simulink model "Project_Sys"  (R2023b)
settings: Solver=ode23t  StartTime=0.0  StopTime=120  RelTol=1e-3
InitFcn:
  | Ts = 0.05;     % Sample time
values from neighbouring files (symbols this model uses):
  B = 4.07973550342    [Project_Dataset.mat]
  Bm = 0.00814489840092    [Project_Dataset.mat]
  g = 9.81    [Project_Dataset.mat]
  JG1 = 0.00809524979335    [Project_Dataset.mat]
  JG2 = 0.148685222339    [Project_Dataset.mat]
  Jm = 0.016692235133    [Project_Dataset.mat]
  Js1 = 0.0287642081421    [Project_Dataset.mat]
  Js2 = 0.0375031699005    [Project_Dataset.mat]
  KT = 0.696639618146    [Project_Dataset.mat]
  L = 0.270608476545    [Project_Dataset.mat]
  La = 0.0921193951949    [Project_Dataset.mat]
  m = 5.3183233869    [Project_Dataset.mat]
  N = 5    [Project_Dataset.mat]
  Ra = 14.3815472022    [Project_Dataset.mat]
libraries: fl_lib x36, nesl_utility x9, ee_lib x3
settings Model: Creator=n01356818  LastModifiedBy=Mystic

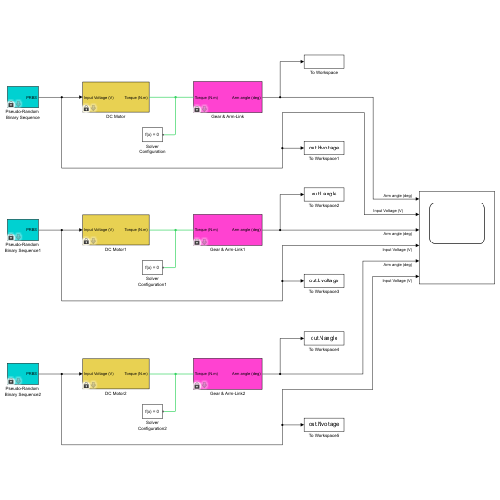
[thumbnail: Simulink's stored preview of the top-level diagram]
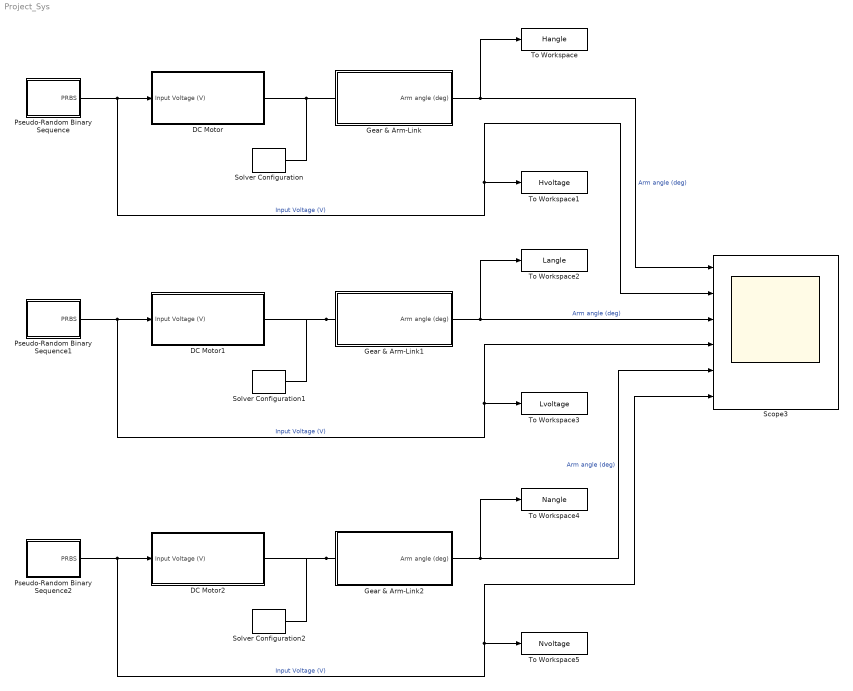
== system Project_Sys ==
  DC Motor : Subsystem  mask(DC Motor){Ra=Ra, La=La, Jm=Jm, Bm=Bm, KT=KT}
      mask prompts: Ra "Armature Resistance - Ra (ohms)"; La "Armature Inductance - La (H)"; Jm "Rotor Inertia - Jm (kg.m^2)"; Bm "Rotor Damping - Bm (N.m.s/rad)"; KT "Torque Constant - KT (N.m/A)"
      mask help: Armature-controlled permanent magnet DC motor with dead-zone nonlinearity.
  DC Motor1 : Subsystem  mask(DC Motor){Ra=Ra, La=La, Jm=Jm, Bm=Bm, KT=KT}
      mask prompts: Ra "Armature Resistance - Ra (ohms)"; La "Armature Inductance - La (H)"; Jm "Rotor Inertia - Jm (kg.m^2)"; Bm "Rotor Damping - Bm (N.m.s/rad)"; KT "Torque Constant - KT (N.m/A)"
      mask help: Armature-controlled permanent magnet DC motor with dead-zone nonlinearity.
  DC Motor2 : Subsystem  mask(DC Motor){Ra=Ra, La=La, Jm=Jm, Bm=Bm, KT=KT}
      mask prompts: Ra "Armature Resistance - Ra (ohms)"; La "Armature Inductance - La (H)"; Jm "Rotor Inertia - Jm (kg.m^2)"; Bm "Rotor Damping - Bm (N.m.s/rad)"; KT "Torque Constant - KT (N.m/A)"
      mask help: Armature-controlled permanent magnet DC motor with dead-zone nonlinearity.
  Gear & Arm-Link : Subsystem  mask(Gear and Arm-link){Js1=Js1, JG1=JG1, Js2=Js2, JG2=JG2, N=N, B=B, m=m, L=L, g=g, noise=1, Ts=Ts}
      mask prompts: Js1 "Drive-side shaft inertia - Js1 (kg.m^2)"; JG1 "Drive-side gear inertia - JG1 (kg.m^2)"; Js2 "Driven-side shaft inertia - Js2 (kg.m^2)"; JG2 "Driven-side gear inertia - JG2 (kg.m^2)"; N "Gear ratio - N (N2/N1)"; B "Damping friction of shaft and arm - B (N.m.s/rad)"; m "Arm mass - m (kg)"; L "Distance of mass center from asix of rotation - L (m)"; g "Gravitational acceleration - g (m/s^2)"; noise "Additive noise (OFF=0, ON=1)"; Ts "Sample time - Ts (sec)"
  Gear & Arm-Link1 : Subsystem  mask(Gear and Arm-link){Js1=Js1, JG1=JG1, Js2=Js2, JG2=JG2, N=N, B=B, m=m, L=L, g=g, noise=1, Ts=Ts}
      mask prompts: Js1 "Drive-side shaft inertia - Js1 (kg.m^2)"; JG1 "Drive-side gear inertia - JG1 (kg.m^2)"; Js2 "Driven-side shaft inertia - Js2 (kg.m^2)"; JG2 "Driven-side gear inertia - JG2 (kg.m^2)"; N "Gear ratio - N (N2/N1)"; B "Damping friction of shaft and arm - B (N.m.s/rad)"; m "Arm mass - m (kg)"; L "Distance of mass center from asix of rotation - L (m)"; g "Gravitational acceleration - g (m/s^2)"; noise "Additive noise (OFF=0, ON=1)"; Ts "Sample time - Ts (sec)"
  Gear & Arm-Link2 : Subsystem  mask(Gear and Arm-link){Js1=Js1, JG1=JG1, Js2=Js2, JG2=JG2, N=N, B=B, m=m, L=L, g=g, noise=0, Ts=Ts}
      mask prompts: Js1 "Drive-side shaft inertia - Js1 (kg.m^2)"; JG1 "Drive-side gear inertia - JG1 (kg.m^2)"; Js2 "Driven-side shaft inertia - Js2 (kg.m^2)"; JG2 "Driven-side gear inertia - JG2 (kg.m^2)"; N "Gear ratio - N (N2/N1)"; B "Damping friction of shaft and arm - B (N.m.s/rad)"; m "Arm mass - m (kg)"; L "Distance of mass center from asix of rotation - L (m)"; g "Gravitational acceleration - g (m/s^2)"; noise "Additive noise (OFF=0, ON=1)"; Ts "Sample time - Ts (sec)"
  Pseudo-Random Binary Sequence : Subsystem  mask(DPRBS){N=250, K=200, A=24}
      mask prompts: N "Number of Sample Points (N)"; K "Switch Constant (K)"; A "Amplitude (A)"
      mask help: Generates a random switching sequence of discrete samples valued at -A and +A.
  Pseudo-Random Binary Sequence1 : Subsystem  mask(DPRBS){N=250, K=200, A=9}
      mask prompts: N "Number of Sample Points (N)"; K "Switch Constant (K)"; A "Amplitude (A)"
      mask help: Generates a random switching sequence of discrete samples valued at -A and +A.
  Pseudo-Random Binary Sequence2 : Subsystem  mask(DPRBS){N=250, K=200, A=24}
      mask prompts: N "Number of Sample Points (N)"; K "Switch Constant (K)"; A "Amplitude (A)"
      mask help: Generates a random switching sequence of discrete samples valued at -A and +A.
  Scope3 : Scope  NumInputPorts=6
  Solver Configuration : nesl_utility/Solver Configuration  PhysicalDomain=network_engine_domain  SubClassName=solver  LeftPortType=input  RightPortType=generic  Tones=[]  Harmonics=[]  SimulateNoise=off  Profile=off  UseLocalSampling=off  EnableSwitchedLinearOptims=on  FrequencyDomain=off  UseCCode=off  RelTol=0.001  AbsTol=0.001  MinStep=1e-09  ToWorkspace=off  RevertToSquareIcSolve=off  NumHomotopyIterations=100  PhasorMode=off  PhasorModeNumHarmonics=1  ConsistencySolver=NEWTON_XTOL_AFTER_FTOL  IndexReductionMethod=DerivativeReplacement  DoDC=off  ResidualTolerance=1e-09  ConsistencyTolSource=GLOBAL  ConsistencyAbsTol=0.001  ConsistencyRelTol=0.001  ConsistencyTolFactor=0.001  UseLocalSolver=off  LocalSolverChoice=NE_BACKWARD_EULER_ADVANCER  ResolveIndetEquations=on  FunctionEvalNumThread=1  LocalSolverSampleTime=0.001  DoFixedCost=off  MaxNonlinIter=3  MaxModeIter=2  ComputeImpulses=off  ImpulseIterations=2  LinearAlgebra=auto  LinearAlgebraNumThread=0  EquationFormulation=NE_TIME_EF  DelaysMemoryBudget=1024  AutomaticFiltering=on  FilteringTimeConstant=0.001  PartitionStorageMethod=AS_NEEDED  PartitionMemoryBudget=1024  PartitionMethod=ROBUST  MultibodyUseLocalSolver=off  MultibodyLocalSolverChoice=ODE1  MultibodyLocalSolverSampleTime=0.001
  Solver Configuration1 : nesl_utility/Solver Configuration  PhysicalDomain=network_engine_domain  SubClassName=solver  LeftPortType=input  RightPortType=generic  Tones=[]  Harmonics=[]  SimulateNoise=off  Profile=off  UseLocalSampling=off  EnableSwitchedLinearOptims=on  FrequencyDomain=off  UseCCode=off  RelTol=0.001  AbsTol=0.001  MinStep=1e-09  ToWorkspace=off  RevertToSquareIcSolve=off  NumHomotopyIterations=100  PhasorMode=off  PhasorModeNumHarmonics=1  ConsistencySolver=NEWTON_XTOL_AFTER_FTOL  IndexReductionMethod=DerivativeReplacement  DoDC=off  ResidualTolerance=1e-09  ConsistencyTolSource=GLOBAL  ConsistencyAbsTol=0.001  ConsistencyRelTol=0.001  ConsistencyTolFactor=0.001  UseLocalSolver=off  LocalSolverChoice=NE_BACKWARD_EULER_ADVANCER  ResolveIndetEquations=on  FunctionEvalNumThread=1  LocalSolverSampleTime=0.001  DoFixedCost=off  MaxNonlinIter=3  MaxModeIter=2  ComputeImpulses=off  ImpulseIterations=2  LinearAlgebra=auto  LinearAlgebraNumThread=0  EquationFormulation=NE_TIME_EF  DelaysMemoryBudget=1024  AutomaticFiltering=on  FilteringTimeConstant=0.001  PartitionStorageMethod=AS_NEEDED  PartitionMemoryBudget=1024  PartitionMethod=ROBUST  MultibodyUseLocalSolver=off  MultibodyLocalSolverChoice=ODE1  MultibodyLocalSolverSampleTime=0.001
  Solver Configuration2 : nesl_utility/Solver Configuration  PhysicalDomain=network_engine_domain  SubClassName=solver  LeftPortType=input  RightPortType=generic  Tones=[]  Harmonics=[]  SimulateNoise=off  Profile=off  UseLocalSampling=off  EnableSwitchedLinearOptims=on  FrequencyDomain=off  UseCCode=off  RelTol=0.001  AbsTol=0.001  MinStep=1e-09  ToWorkspace=off  RevertToSquareIcSolve=off  NumHomotopyIterations=100  PhasorMode=off  PhasorModeNumHarmonics=1  ConsistencySolver=NEWTON_XTOL_AFTER_FTOL  IndexReductionMethod=DerivativeReplacement  DoDC=off  ResidualTolerance=1e-09  ConsistencyTolSource=GLOBAL  ConsistencyAbsTol=0.001  ConsistencyRelTol=0.001  ConsistencyTolFactor=0.001  UseLocalSolver=off  LocalSolverChoice=NE_BACKWARD_EULER_ADVANCER  ResolveIndetEquations=on  FunctionEvalNumThread=1  LocalSolverSampleTime=0.001  DoFixedCost=off  MaxNonlinIter=3  MaxModeIter=2  ComputeImpulses=off  ImpulseIterations=2  LinearAlgebra=auto  LinearAlgebraNumThread=0  EquationFormulation=NE_TIME_EF  DelaysMemoryBudget=1024  AutomaticFiltering=on  FilteringTimeConstant=0.001  PartitionStorageMethod=AS_NEEDED  PartitionMemoryBudget=1024  PartitionMethod=ROBUST  MultibodyUseLocalSolver=off  MultibodyLocalSolverChoice=ODE1  MultibodyLocalSolverSampleTime=0.001
  To Workspace : ToWorkspace  VariableName=Hangle  SampleTime=Ts
  To Workspace1 : ToWorkspace  VariableName=Hvoltage  SampleTime=Ts
  To Workspace2 : ToWorkspace  VariableName=Langle  SampleTime=Ts
  To Workspace3 : ToWorkspace  VariableName=Lvoltage  SampleTime=Ts
  To Workspace4 : ToWorkspace  VariableName=Nangle  SampleTime=Ts
  To Workspace5 : ToWorkspace  VariableName=Nvoltage  SampleTime=Ts
  wires:
  Pseudo-Random Binary Sequence/1(PRBS) -> Scope3/2, To Workspace1/1, DC Motor/1(Input Voltage (V))  "Input Voltage (V)"
  Gear & Arm-Link/1(Arm angle (deg)) -> Scope3/1, To Workspace/1  "Arm angle (deg)"
  Pseudo-Random Binary Sequence1/1(PRBS) -> Scope3/4, To Workspace3/1, DC Motor1/1(Input Voltage (V))  "Input Voltage (V)"
  Gear & Arm-Link1/1(Arm angle (deg)) -> Scope3/3, To Workspace2/1  "Arm angle (deg)"
  Pseudo-Random Binary Sequence2/1(PRBS) -> Scope3/6, To Workspace5/1, DC Motor2/1(Input Voltage (V))  "Input Voltage (V)"
  Gear & Arm-Link2/1(Arm angle (deg)) -> Scope3/5, To Workspace4/1  "Arm angle (deg)"
  connections:
  DC Motor/RConn1 -- Solver Configuration/RConn1 -- Gear & Arm-Link/LConn1
  Gear & Arm-Link1/LConn1 -- DC Motor1/RConn1 -- Solver Configuration1/RConn1
  Gear & Arm-Link2/LConn1 -- DC Motor2/RConn1 -- Solver Configuration2/RConn1

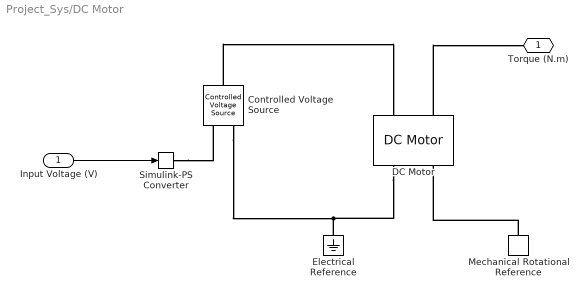
== system Project_Sys/DC Motor ==
  Input Voltage (V) : Inport
  Controlled Voltage Source : fl_lib/Electrical/Electrical Sources/Controlled Voltage Source
  DC Motor : ee_lib/Electromechanical/Brushed Motors/DC Motor  field_option=ee.enum.field_option.pm  Rf=100 Ohm  Lf=1 H  Laf=0.15 H  If0=0 A  parameterization=ee.enum.dcparam_option.circuit_param  Ra=Ra Ohm  La=La H  emf_or_torque=ee.enum.emf_or_torque.ki  Kv=0.4 V*s/rad  Ki=KT N*m/A  T_stall=0.24e-3 N*m  w_max=19100 rpm  w_rated=15000 rpm  P_rated=0.08 W  V_rated=1.5 V  lam_param=ee.enum.lam_param.damping  i_noload=0 A  V_i_noload=1.5 V  J=Jm kg*m^2  lam=Bm N*m*s/rad  speed0=0 rpm  enable_fault_armature=simscape.enum.onoff.off  rev_faulted=1 / 3  G_faulted_armature=1e-5 S  fault_trigger_armature=ee.enum.faults.faultTrigger.temporal  t_fault_armature=1 s  max_permissible_current_armature=inf A  t_fail_on_current_armature=1 s  enable_fault_field=simscape.enum.onoff.off  G_faulted_field=1e-5 S  fault_trigger_field=ee.enum.faults.faultTrigger.temporal  t_fault_field=1 s  max_permissible_current_field=inf A  t_fail_on_current_field=1 s  fault_action=simscape.enum.assert.action.none  alpha=3.93e-3 1/K  Tmeas=25 degC  thermal_mass=100 J/K  initial_temperature=25 degC
  Electrical Reference : fl_lib/Electrical/Electrical Elements/Electrical Reference
  Mechanical Rotational Reference : fl_lib/Mechanical/Rotational Elements/Mechanical Rotational Reference
  Simulink-PS Converter : nesl_utility/Simulink-PS Converter  PhysicalDomain=network_engine_domain  SubClassName=ps_input  LeftPortType=input  RightPortType=output  PseudoPeriodic=off  Frequencies=[]  NoiseDistribution=none  NoiseParameters=[]  Unit=1  AffineConversion=off  FilteringAndDerivatives=provide  SimscapeFilterOrder=1  InputFilterTimeConstant=0.001  UdotUserProvided=0
  Torque (N.m) : PMIOPort  Side=Right
  wires:
  Input Voltage (V)/1 -> Simulink-PS Converter/1
  connections:
  DC Motor/RConn1 -- Controlled Voltage Source/RConn2 -- Electrical Reference/LConn1
  Simulink-PS Converter/RConn1 -- Controlled Voltage Source/RConn1
  Controlled Voltage Source/LConn1 -- DC Motor/LConn1
  Mechanical Rotational Reference/LConn1 -- DC Motor/RConn2
  DC Motor/LConn2 -- Torque (N.m)/RConn1

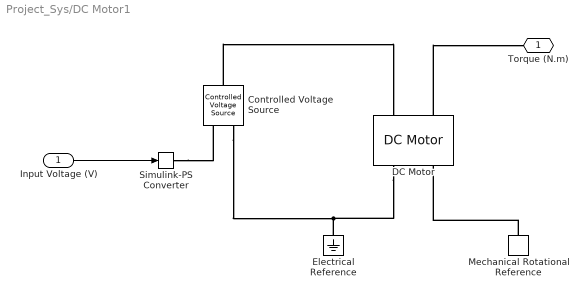
== system Project_Sys/DC Motor1 ==
  Input Voltage (V) : Inport
  Controlled Voltage Source : fl_lib/Electrical/Electrical Sources/Controlled Voltage Source
  DC Motor : ee_lib/Electromechanical/Brushed Motors/DC Motor  field_option=ee.enum.field_option.pm  Rf=100 Ohm  Lf=1 H  Laf=0.15 H  If0=0 A  parameterization=ee.enum.dcparam_option.circuit_param  Ra=Ra Ohm  La=La H  emf_or_torque=ee.enum.emf_or_torque.ki  Kv=0.4 V*s/rad  Ki=KT N*m/A  T_stall=0.24e-3 N*m  w_max=19100 rpm  w_rated=15000 rpm  P_rated=0.08 W  V_rated=1.5 V  lam_param=ee.enum.lam_param.damping  i_noload=0 A  V_i_noload=1.5 V  J=Jm kg*m^2  lam=Bm N*m*s/rad  speed0=0 rpm  enable_fault_armature=simscape.enum.onoff.off  rev_faulted=1 / 3  G_faulted_armature=1e-5 S  fault_trigger_armature=ee.enum.faults.faultTrigger.temporal  t_fault_armature=1 s  max_permissible_current_armature=inf A  t_fail_on_current_armature=1 s  enable_fault_field=simscape.enum.onoff.off  G_faulted_field=1e-5 S  fault_trigger_field=ee.enum.faults.faultTrigger.temporal  t_fault_field=1 s  max_permissible_current_field=inf A  t_fail_on_current_field=1 s  fault_action=simscape.enum.assert.action.none  alpha=3.93e-3 1/K  Tmeas=25 degC  thermal_mass=100 J/K  initial_temperature=25 degC
  Electrical Reference : fl_lib/Electrical/Electrical Elements/Electrical Reference
  Mechanical Rotational Reference : fl_lib/Mechanical/Rotational Elements/Mechanical Rotational Reference
  Simulink-PS Converter : nesl_utility/Simulink-PS Converter  PhysicalDomain=network_engine_domain  SubClassName=ps_input  LeftPortType=input  RightPortType=output  PseudoPeriodic=off  Frequencies=[]  NoiseDistribution=none  NoiseParameters=[]  Unit=1  AffineConversion=off  FilteringAndDerivatives=provide  SimscapeFilterOrder=1  InputFilterTimeConstant=0.001  UdotUserProvided=0
  Torque (N.m) : PMIOPort  Side=Right
  wires:
  Input Voltage (V)/1 -> Simulink-PS Converter/1
  connections:
  DC Motor/RConn1 -- Controlled Voltage Source/RConn2 -- Electrical Reference/LConn1
  Simulink-PS Converter/RConn1 -- Controlled Voltage Source/RConn1
  Controlled Voltage Source/LConn1 -- DC Motor/LConn1
  Mechanical Rotational Reference/LConn1 -- DC Motor/RConn2
  DC Motor/LConn2 -- Torque (N.m)/RConn1

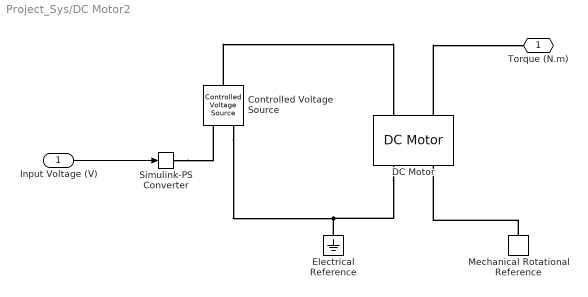
== system Project_Sys/DC Motor2 ==
  Input Voltage (V) : Inport
  Controlled Voltage Source : fl_lib/Electrical/Electrical Sources/Controlled Voltage Source
  DC Motor : ee_lib/Electromechanical/Brushed Motors/DC Motor  field_option=ee.enum.field_option.pm  Rf=100 Ohm  Lf=1 H  Laf=0.15 H  If0=0 A  parameterization=ee.enum.dcparam_option.circuit_param  Ra=Ra Ohm  La=La H  emf_or_torque=ee.enum.emf_or_torque.ki  Kv=0.4 V*s/rad  Ki=KT N*m/A  T_stall=0.24e-3 N*m  w_max=19100 rpm  w_rated=15000 rpm  P_rated=0.08 W  V_rated=1.5 V  lam_param=ee.enum.lam_param.damping  i_noload=0 A  V_i_noload=1.5 V  J=Jm kg*m^2  lam=Bm N*m*s/rad  speed0=0 rpm  enable_fault_armature=simscape.enum.onoff.off  rev_faulted=1 / 3  G_faulted_armature=1e-5 S  fault_trigger_armature=ee.enum.faults.faultTrigger.temporal  t_fault_armature=1 s  max_permissible_current_armature=inf A  t_fail_on_current_armature=1 s  enable_fault_field=simscape.enum.onoff.off  G_faulted_field=1e-5 S  fault_trigger_field=ee.enum.faults.faultTrigger.temporal  t_fault_field=1 s  max_permissible_current_field=inf A  t_fail_on_current_field=1 s  fault_action=simscape.enum.assert.action.none  alpha=3.93e-3 1/K  Tmeas=25 degC  thermal_mass=100 J/K  initial_temperature=25 degC
  Electrical Reference : fl_lib/Electrical/Electrical Elements/Electrical Reference
  Mechanical Rotational Reference : fl_lib/Mechanical/Rotational Elements/Mechanical Rotational Reference
  Simulink-PS Converter : nesl_utility/Simulink-PS Converter  PhysicalDomain=network_engine_domain  SubClassName=ps_input  LeftPortType=input  RightPortType=output  PseudoPeriodic=off  Frequencies=[]  NoiseDistribution=none  NoiseParameters=[]  Unit=1  AffineConversion=off  FilteringAndDerivatives=provide  SimscapeFilterOrder=1  InputFilterTimeConstant=0.001  UdotUserProvided=0
  Torque (N.m) : PMIOPort  Side=Right
  wires:
  Input Voltage (V)/1 -> Simulink-PS Converter/1
  connections:
  DC Motor/RConn1 -- Controlled Voltage Source/RConn2 -- Electrical Reference/LConn1
  Simulink-PS Converter/RConn1 -- Controlled Voltage Source/RConn1
  Controlled Voltage Source/LConn1 -- DC Motor/LConn1
  Mechanical Rotational Reference/LConn1 -- DC Motor/RConn2
  DC Motor/LConn2 -- Torque (N.m)/RConn1

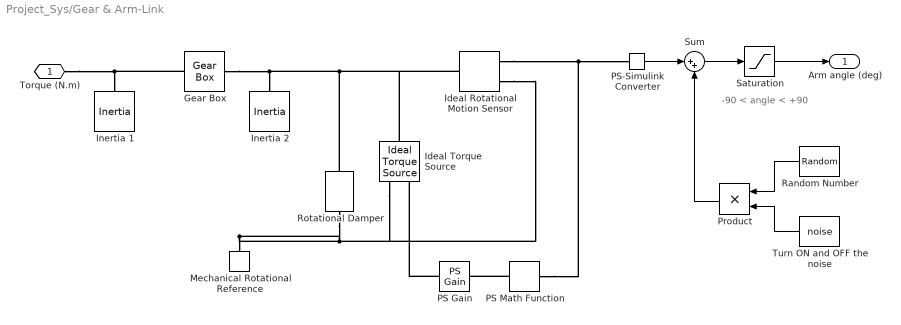
== system Project_Sys/Gear & Arm-Link ==
  note: -90 < angle < +90
  Gear Box : fl_lib/Mechanical/Mechanisms/Gear Box  ratio=N  t_in_specify=off  t_in_priority=None  t_in=0 N*m  t_in_nominal_specify=off  t_in_nominal_unit=N*m  t_in_nominal_value=1  t_out_specify=off  t_out_priority=None  t_out=0 N*m  t_out_nominal_specify=off  t_out_nominal_unit=N*m  t_out_nominal_value=1
  Ideal Rotational Motion Sensor : fl_lib/Mechanical/Mechanical Sensors/Ideal Rotational Motion Sensor  reference=foundation.enum.MeasurementReference.difference  acceleration_port=false  velocity_port=false  position_port=true  wrap_angle=false  offset=0 rad
      settings: InternalSimscapePortConfiguration="{\"Bottom\":[],\"Left\":[{\"id\":\"R\",\"label\":\"R\",\"type\":\"foundation.mechanical.rotational.rotational\"}],\"Right\":[{\"id\":\"C\",\"label\":\"C\",\"type\":\"foundation.mechanical.rotational.rotational\"},{\"id\":\"A\",\"label\":\"A\",\"type\":\"output\"}],\"Top\":[]}"
  Ideal Torque Source : fl_lib/Mechanical/Mechanical Sources/Ideal Torque Source
  Inertia 1 : fl_lib/Mechanical/Rotational Elements/Inertia  inertia=Js1+JG1 kg*m^2  num_ports=foundation.enum.numPorts2.one  w_specify=off  w_priority=High  w=0 rad/s  w_nominal_specify=off  w_nominal_unit=rad/s  w_nominal_value=1  t_specify=off  t_priority=None  t=0 N*m  t_nominal_specify=off  t_nominal_unit=N*m  t_nominal_value=1
  Inertia 2 : fl_lib/Mechanical/Rotational Elements/Inertia  inertia=Js2+JG2 kg*m^2  num_ports=foundation.enum.numPorts2.one  w_specify=off  w_priority=High  w=0 rad/s  w_nominal_specify=off  w_nominal_unit=rad/s  w_nominal_value=1  t_specify=off  t_priority=None  t=0 N*m  t_nominal_specify=off  t_nominal_unit=N*m  t_nominal_value=1
  Mechanical Rotational Reference : fl_lib/Mechanical/Rotational Elements/Mechanical Rotational Reference
  PS Gain : fl_lib/Physical Signals/Functions/PS Gain  gain=-m*g*L
  PS Math Function : fl_lib/Physical Signals/Functions/PS Math Function  fcn_choice=foundation.enum.math_function.sin  v=1
  PS-Simulink Converter : nesl_utility/PS-Simulink Converter  PhysicalDomain=network_engine_domain  SubClassName=ps_output  LeftPortType=input  RightPortType=output  PseudoPeriodic=off  Frequencies=[]  VectorFormat=inherit  Unit=deg  AffineConversion=off
  Product : Product
  Random Number : RandomNumber  Seed=randi([0 100],1,1)  SampleTime=0.1*Ts
  Rotational Damper : fl_lib/Mechanical/Rotational Elements/Rotational Damper  D=B N*m*s/rad  w_specify=off  w_priority=None  w=0 rad/s  w_nominal_specify=off  w_nominal_unit=rad/s  w_nominal_value=1  t_specify=off  t_priority=None  t=0 N*m  t_nominal_specify=off  t_nominal_unit=N*m  t_nominal_value=1
  Saturation : Saturate  UpperLimit=90  LowerLimit=-90
  Sum : Sum  Inputs=|++
  Turn ON and OFF the noise : Constant  Value=noise  SampleTime=0.1*Ts
  Torque (N.m) : PMIOPort  Side=Left
  Arm angle (deg) : Outport
  wires:
  Turn ON and OFF the noise/1 -> Product/2
  Random Number/1 -> Product/1
  Product/1 -> Sum/2
  PS-Simulink Converter/1 -> Sum/1
  Sum/1 -> Saturation/1
  Saturation/1 -> Arm angle (deg)/1
  connections:
  PS Gain/RConn1 -- Ideal Torque Source/RConn1
  Ideal Rotational Motion Sensor/RConn2 -- PS Math Function/LConn1 -- PS-Simulink Converter/LConn1
  Mechanical Rotational Reference/LConn1 -- Ideal Rotational Motion Sensor/RConn1 -- Ideal Torque Source/RConn2 -- Rotational Damper/RConn1
  PS Math Function/RConn1 -- PS Gain/LConn1
  Gear Box/RConn1 -- Ideal Rotational Motion Sensor/LConn1 -- Ideal Torque Source/LConn1 -- Rotational Damper/LConn1 -- Inertia 2/LConn1
  Gear Box/LConn1 -- Torque (N.m)/RConn1 -- Inertia 1/LConn1

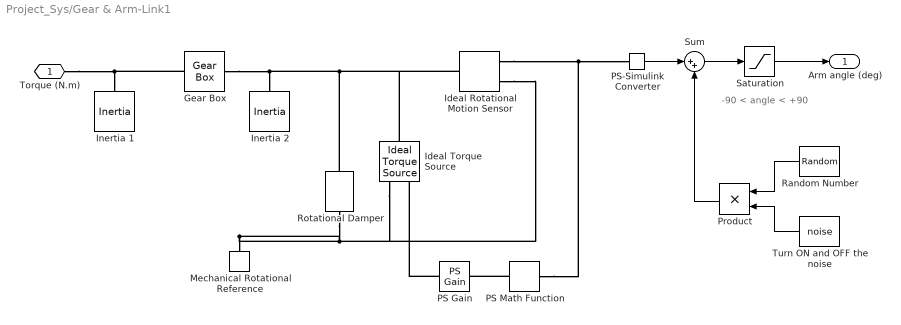
== system Project_Sys/Gear & Arm-Link1 ==
  note: -90 < angle < +90
  Gear Box : fl_lib/Mechanical/Mechanisms/Gear Box  ratio=N  t_in_specify=off  t_in_priority=None  t_in=0 N*m  t_in_nominal_specify=off  t_in_nominal_unit=N*m  t_in_nominal_value=1  t_out_specify=off  t_out_priority=None  t_out=0 N*m  t_out_nominal_specify=off  t_out_nominal_unit=N*m  t_out_nominal_value=1
  Ideal Rotational Motion Sensor : fl_lib/Mechanical/Mechanical Sensors/Ideal Rotational Motion Sensor  reference=foundation.enum.MeasurementReference.difference  acceleration_port=false  velocity_port=false  position_port=true  wrap_angle=false  offset=0 rad
      settings: InternalSimscapePortConfiguration="{\"Bottom\":[],\"Left\":[{\"id\":\"R\",\"label\":\"R\",\"type\":\"foundation.mechanical.rotational.rotational\"}],\"Right\":[{\"id\":\"C\",\"label\":\"C\",\"type\":\"foundation.mechanical.rotational.rotational\"},{\"id\":\"A\",\"label\":\"A\",\"type\":\"output\"}],\"Top\":[]}"
  Ideal Torque Source : fl_lib/Mechanical/Mechanical Sources/Ideal Torque Source
  Inertia 1 : fl_lib/Mechanical/Rotational Elements/Inertia  inertia=Js1+JG1 kg*m^2  num_ports=foundation.enum.numPorts2.one  w_specify=off  w_priority=High  w=0 rad/s  w_nominal_specify=off  w_nominal_unit=rad/s  w_nominal_value=1  t_specify=off  t_priority=None  t=0 N*m  t_nominal_specify=off  t_nominal_unit=N*m  t_nominal_value=1
  Inertia 2 : fl_lib/Mechanical/Rotational Elements/Inertia  inertia=Js2+JG2 kg*m^2  num_ports=foundation.enum.numPorts2.one  w_specify=off  w_priority=High  w=0 rad/s  w_nominal_specify=off  w_nominal_unit=rad/s  w_nominal_value=1  t_specify=off  t_priority=None  t=0 N*m  t_nominal_specify=off  t_nominal_unit=N*m  t_nominal_value=1
  Mechanical Rotational Reference : fl_lib/Mechanical/Rotational Elements/Mechanical Rotational Reference
  PS Gain : fl_lib/Physical Signals/Functions/PS Gain  gain=-m*g*L
  PS Math Function : fl_lib/Physical Signals/Functions/PS Math Function  fcn_choice=foundation.enum.math_function.sin  v=1
  PS-Simulink Converter : nesl_utility/PS-Simulink Converter  PhysicalDomain=network_engine_domain  SubClassName=ps_output  LeftPortType=input  RightPortType=output  PseudoPeriodic=off  Frequencies=[]  VectorFormat=inherit  Unit=deg  AffineConversion=off
  Product : Product
  Random Number : RandomNumber  Seed=randi([0 100],1,1)  SampleTime=0.1*Ts
  Rotational Damper : fl_lib/Mechanical/Rotational Elements/Rotational Damper  D=B N*m*s/rad  w_specify=off  w_priority=None  w=0 rad/s  w_nominal_specify=off  w_nominal_unit=rad/s  w_nominal_value=1  t_specify=off  t_priority=None  t=0 N*m  t_nominal_specify=off  t_nominal_unit=N*m  t_nominal_value=1
  Saturation : Saturate  UpperLimit=90  LowerLimit=-90
  Sum : Sum  Inputs=|++
  Turn ON and OFF the noise : Constant  Value=noise  SampleTime=0.1*Ts
  Torque (N.m) : PMIOPort  Side=Left
  Arm angle (deg) : Outport
  wires:
  Turn ON and OFF the noise/1 -> Product/2
  Random Number/1 -> Product/1
  Product/1 -> Sum/2
  PS-Simulink Converter/1 -> Sum/1
  Sum/1 -> Saturation/1
  Saturation/1 -> Arm angle (deg)/1
  connections:
  PS Gain/RConn1 -- Ideal Torque Source/RConn1
  Ideal Rotational Motion Sensor/RConn2 -- PS Math Function/LConn1 -- PS-Simulink Converter/LConn1
  Mechanical Rotational Reference/LConn1 -- Ideal Rotational Motion Sensor/RConn1 -- Ideal Torque Source/RConn2 -- Rotational Damper/RConn1
  PS Math Function/RConn1 -- PS Gain/LConn1
  Gear Box/RConn1 -- Ideal Rotational Motion Sensor/LConn1 -- Ideal Torque Source/LConn1 -- Rotational Damper/LConn1 -- Inertia 2/LConn1
  Gear Box/LConn1 -- Torque (N.m)/RConn1 -- Inertia 1/LConn1

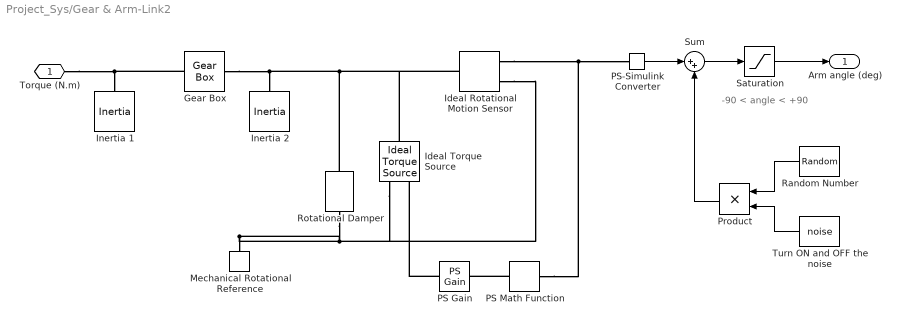
== system Project_Sys/Gear & Arm-Link2 ==
  note: -90 < angle < +90
  Gear Box : fl_lib/Mechanical/Mechanisms/Gear Box  ratio=N  t_in_specify=off  t_in_priority=None  t_in=0 N*m  t_in_nominal_specify=off  t_in_nominal_unit=N*m  t_in_nominal_value=1  t_out_specify=off  t_out_priority=None  t_out=0 N*m  t_out_nominal_specify=off  t_out_nominal_unit=N*m  t_out_nominal_value=1
  Ideal Rotational Motion Sensor : fl_lib/Mechanical/Mechanical Sensors/Ideal Rotational Motion Sensor  reference=foundation.enum.MeasurementReference.difference  acceleration_port=false  velocity_port=false  position_port=true  wrap_angle=false  offset=0 rad
      settings: InternalSimscapePortConfiguration="{\"Bottom\":[],\"Left\":[{\"id\":\"R\",\"label\":\"R\",\"type\":\"foundation.mechanical.rotational.rotational\"}],\"Right\":[{\"id\":\"C\",\"label\":\"C\",\"type\":\"foundation.mechanical.rotational.rotational\"},{\"id\":\"A\",\"label\":\"A\",\"type\":\"output\"}],\"Top\":[]}"
  Ideal Torque Source : fl_lib/Mechanical/Mechanical Sources/Ideal Torque Source
  Inertia 1 : fl_lib/Mechanical/Rotational Elements/Inertia  inertia=Js1+JG1 kg*m^2  num_ports=foundation.enum.numPorts2.one  w_specify=off  w_priority=High  w=0 rad/s  w_nominal_specify=off  w_nominal_unit=rad/s  w_nominal_value=1  t_specify=off  t_priority=None  t=0 N*m  t_nominal_specify=off  t_nominal_unit=N*m  t_nominal_value=1
  Inertia 2 : fl_lib/Mechanical/Rotational Elements/Inertia  inertia=Js2+JG2 kg*m^2  num_ports=foundation.enum.numPorts2.one  w_specify=off  w_priority=High  w=0 rad/s  w_nominal_specify=off  w_nominal_unit=rad/s  w_nominal_value=1  t_specify=off  t_priority=None  t=0 N*m  t_nominal_specify=off  t_nominal_unit=N*m  t_nominal_value=1
  Mechanical Rotational Reference : fl_lib/Mechanical/Rotational Elements/Mechanical Rotational Reference
  PS Gain : fl_lib/Physical Signals/Functions/PS Gain  gain=-m*g*L
  PS Math Function : fl_lib/Physical Signals/Functions/PS Math Function  fcn_choice=foundation.enum.math_function.sin  v=1
  PS-Simulink Converter : nesl_utility/PS-Simulink Converter  PhysicalDomain=network_engine_domain  SubClassName=ps_output  LeftPortType=input  RightPortType=output  PseudoPeriodic=off  Frequencies=[]  VectorFormat=inherit  Unit=deg  AffineConversion=off
  Product : Product
  Random Number : RandomNumber  Seed=randi([0 100],1,1)  SampleTime=0.1*Ts
  Rotational Damper : fl_lib/Mechanical/Rotational Elements/Rotational Damper  D=B N*m*s/rad  w_specify=off  w_priority=None  w=0 rad/s  w_nominal_specify=off  w_nominal_unit=rad/s  w_nominal_value=1  t_specify=off  t_priority=None  t=0 N*m  t_nominal_specify=off  t_nominal_unit=N*m  t_nominal_value=1
  Saturation : Saturate  UpperLimit=90  LowerLimit=-90
  Sum : Sum  Inputs=|++
  Turn ON and OFF the noise : Constant  Value=noise  SampleTime=0.1*Ts
  Torque (N.m) : PMIOPort  Side=Left
  Arm angle (deg) : Outport
  wires:
  Turn ON and OFF the noise/1 -> Product/2
  Random Number/1 -> Product/1
  Product/1 -> Sum/2
  PS-Simulink Converter/1 -> Sum/1
  Sum/1 -> Saturation/1
  Saturation/1 -> Arm angle (deg)/1
  connections:
  PS Gain/RConn1 -- Ideal Torque Source/RConn1
  Ideal Rotational Motion Sensor/RConn2 -- PS Math Function/LConn1 -- PS-Simulink Converter/LConn1
  Mechanical Rotational Reference/LConn1 -- Ideal Rotational Motion Sensor/RConn1 -- Ideal Torque Source/RConn2 -- Rotational Damper/RConn1
  PS Math Function/RConn1 -- PS Gain/LConn1
  Gear Box/RConn1 -- Ideal Rotational Motion Sensor/LConn1 -- Ideal Torque Source/LConn1 -- Rotational Damper/LConn1 -- Inertia 2/LConn1
  Gear Box/LConn1 -- Torque (N.m)/RConn1 -- Inertia 1/LConn1

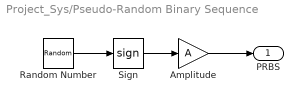
== system Project_Sys/Pseudo-Random Binary Sequence ==
  Amplitude : Gain  Gain=A
  Random Number : RandomNumber  Seed=randi([0 100],1,1)  SampleTime=10*K/N
  Sign : Signum
  PRBS : Outport
  wires:
  Sign/1 -> Amplitude/1
  Random Number/1 -> Sign/1
  Amplitude/1 -> PRBS/1

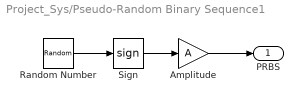
== system Project_Sys/Pseudo-Random Binary Sequence1 ==
  Amplitude : Gain  Gain=A
  Random Number : RandomNumber  Seed=randi([0 100],1,1)  SampleTime=10*K/N
  Sign : Signum
  PRBS : Outport
  wires:
  Sign/1 -> Amplitude/1
  Random Number/1 -> Sign/1
  Amplitude/1 -> PRBS/1

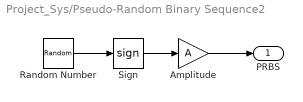
== system Project_Sys/Pseudo-Random Binary Sequence2 ==
  Amplitude : Gain  Gain=A
  Random Number : RandomNumber  Seed=randi([0 100],1,1)  SampleTime=10*K/N
  Sign : Signum
  PRBS : Outport
  wires:
  Sign/1 -> Amplitude/1
  Random Number/1 -> Sign/1
  Amplitude/1 -> PRBS/1
